simulink model "robot_locomotion_SL_VelTurn"  (R2026a)
settings: Solver=VariableStepAuto  StopTime=tEnd  AbsTol=1e-3  EnableMultiTasking=on
values from neighbouring files (symbols this model uses):
  alb = 0.1    [TunedPIDworkspace.mat]
  albv = 0.2    [TunedPIDworkspace.mat]
  altr = 0.3    [TunedPIDworkspace.mat]
  battery_mass = 0.167    [TunedPIDworkspace.mat]    (also in robot_script_RL_Vel.m; robot_script_RL_VelDual.m; robot_script_RL_VelTurn.m)
  battery_z_pos = -0.035    [TunedPIDworkspace.mat]    (also in robot_script_RL_Vel.m; robot_script_RL_VelDual.m; robot_script_RL_VelTurn.m)
  bypass_b = 0    [TunedPIDworkspace.mat]
  bypass_bi = 0    [TunedPIDworkspace.mat]
  bypass_bp = 1    [TunedPIDworkspace.mat]
  bypass_bv = 0    [TunedPIDworkspace.mat]
  fftr = 0    [TunedPIDworkspace.mat]
  ffv = 7    [TunedPIDworkspace.mat]
  Kpb = -0.55    [TunedPIDworkspace.mat]
  kpbp = 1.4    [TunedPIDworkspace.mat]
  Kpbv = -2    [TunedPIDworkspace.mat]
  Kptr = 1    [TunedPIDworkspace.mat]
  kpv = 10    [TunedPIDworkspace.mat]
  mass_left = 0.325    [TunedPIDworkspace.mat]    (also in robot_script_RL_Vel.m; robot_script_RL_VelDual.m; robot_script_RL_VelTurn.m)
  maxV = 10    [TunedPIDworkspace.mat]    (also in robot_script_RL_Vel.m; robot_script_RL_VelDual.m; robot_script_RL_VelTurn.m)
  motor_z_pos = -0.022    [TunedPIDworkspace.mat]    (also in robot_script_RL_Vel.m; robot_script_RL_VelDual.m; robot_script_RL_VelTurn.m)
  N = size(data, 1)    [robot_script_PIDvsNN.m]
  pcb_mass = 0.098    [TunedPIDworkspace.mat]    (also in robot_script_RL_Vel.m; robot_script_RL_VelDual.m; robot_script_RL_VelTurn.m)
  robot_width = 0.15    [TunedPIDworkspace.mat]    (also in robot_script_RL_Vel.m; robot_script_RL_VelDual.m; robot_script_RL_VelTurn.m)
  s = tf('s')    [robot_script_PIDvsNN.m]    (also in robot_script_RL_Vel.m; robot_script_RL_VelDual.m; robot_script_RL_VelTurn.m)
  taubd = 0.15    [TunedPIDworkspace.mat]
  taubi = 0.1    [TunedPIDworkspace.mat]
  taubii = 0.1    [TunedPIDworkspace.mat]
  taubp = 100000    [TunedPIDworkspace.mat]
  taubvd = 0.6    [TunedPIDworkspace.mat]
  taubvf = 0.01    [TunedPIDworkspace.mat]
  taubvi = 1    [TunedPIDworkspace.mat]
  tautrd = 0.22    [TunedPIDworkspace.mat]
  tautri = 0.1    [TunedPIDworkspace.mat]
  tauvi = 0.043    [TunedPIDworkspace.mat]
  vel_bp = 0.4    [TunedPIDworkspace.mat]
  Y = 20*log10(abs(fft(data)))    [robot_script_PIDvsNN.m]
undefined symbols (not defined in the file or in its folder): net_trained, X, Z
libraries: sm_lib x39, fl_lib x16, nesl_utility x15, ee_lib x4, dlconvfclib x3, dlactivationlib x3, dlutilitylib x1, sharedtransform x1
(part 1 of 2)
settings Model: Creator=chr  LastModifiedBy=emil
settings SimscapeCC: SimscapeNominalValues="[{\"value\":\"1\",\"unit\":\"A\"},{\"value\":\"1\",\"unit\":\"bar\"},{\"value\":\"1\",\"unit\":\"cm^2\"},{\"value\":\"1\",\"unit\":\"cm^3/s\"},{\"value\":\"1\",\"unit\":\"kJ/kg\"},{\"value\":\"1\",\"unit\":\"kW\"},{\"value\":\"1\",\"unit\":\"l\"},{\"value\":\"1\",\"unit\":\"N\"},{\"value\":\"1\",\"unit\":\"N*m\"},{\"value\":\"1\",\"unit\":\"V\"}]"  SimscapeLogSimulationStatistics=on
settings ExplorerConfigSet: SimMechanicsOpenEditorOnUpdate=off
settings ExplorerConfigSet: InternalSimMechanicsExplorerSettings=|
  | <ExplorerConfiguration>
  | 
  |   <canonicalview>default</canonicalview>
  | 
  |   <TilePanel>
  |     <TileInfo>
  |       <Tiles Columns="1" Count="1" Height="704" Rows="1" Width="1078">
  |         <Row Weight="1"/>
  |         <Column Weight="1"/>
  |         <Tile Height="1" Width="1" X="0" Y="0"/>
  |       </Tiles>
  |     </TileInfo>
  |     <SceneInfo>
  |       <SceneViewer>
  |         <IsThisViewStd>
  |           <IsStandardView>off</IsStandardView>
  |           <StandardViewName>Front</StandardViewName>
  |         </IsThisViewStd>
  |         <BGColor>
  |           <R>1</R>
  |           <G>1</G>
  |           <B>1</B>
  |           <A>1</A>
  |         </BGColor>
  |         <Camera>
  |           <DoPerspective>off</DoPerspective>
  |           <Position>
  |             <X>48.876368132250072</X>
  |             <Y>-48.984454841396008</Y>
  |             <Z>49.183620508129628</Z>
  |           </Position>
  |           <Center>
  |             <X>-0.11465636167667981</X>
  |             <Y>0.006569652530743042</Y>
  |             <Z>0.19259601420287537</Z>
  |           </Center>
  |           <Up>
  |             <X>-0.40824829046386307</X>
  |             <Y>0.40824829046386307</Y>
  |             <Z>0.81649658092772615</Z>
  |           </Up>
  |           <XLim>2.040943635816892</XLim>
  |           <YLim>2.040943635816892</YLim>
  |           <ViewLimDist>0.01</ViewLimDist>
  |         </Camera>
  |       </SceneViewer>
  |     </SceneInfo>
  |   </TilePanel>
  | 
  |   <MechEditorPanel>
  |     <GfxPanelCameraMap/>
  |     <Cameras/>
  |     <VideoCreator>
  |       <IncludeTiles>All</IncludeTiles>
  |       <IncludeTime>on</IncludeTime>
  |       <IncludeWorldFrame>off</IncludeWorldFrame>
  |       <PlaybackSpeedRatio>1</PlaybackSpeedRatio>
  |       <FrameRate>30</FrameRate>
  |       <FrameSize>auto</FrameSize>
  |       <VideoFormat>UncompressedAVI</VideoFormat>
  |     </VideoCreator>
  |   </MechEditorPanel>
  | 
  |   <PlaybackSettings>
  |     <PlaybackSpeedFactor>4</PlaybackSpeedFactor>
  |   </PlaybackSettings>
  | 
  | </ExplorerConfiguration>

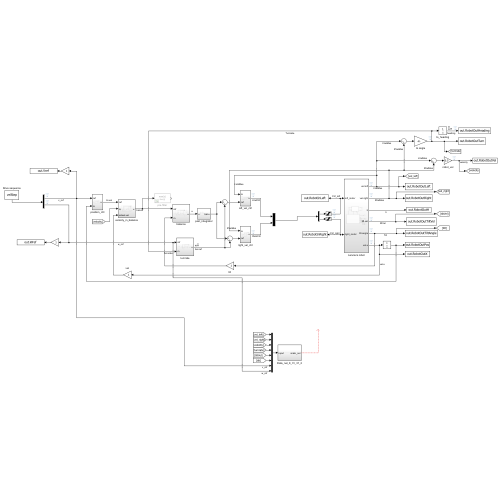
[thumbnail: Simulink's stored preview of the top-level diagram]
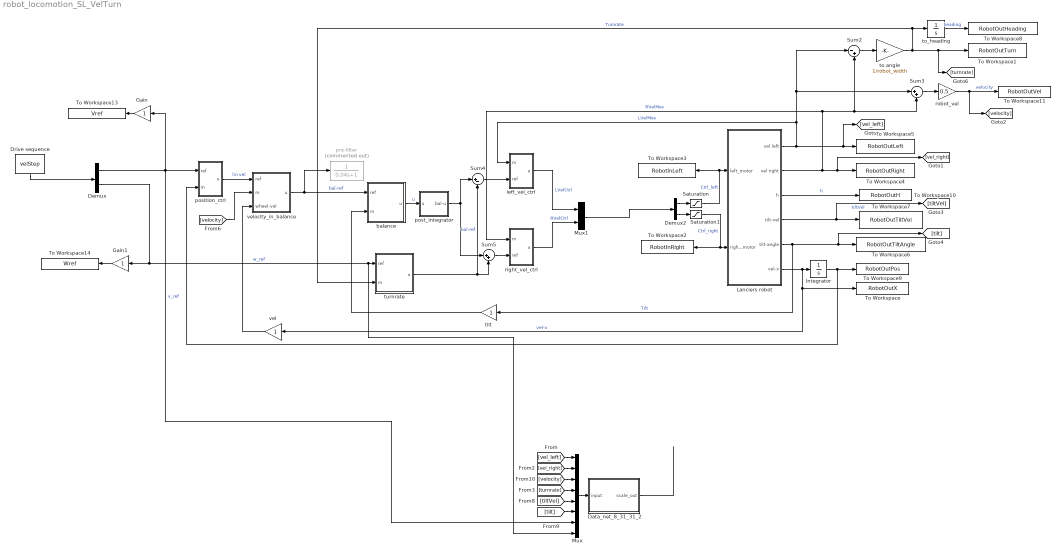
== system robot_locomotion_SL_VelTurn ==
  Data_net_8_31_31_2 : Subsystem
  Demux : Demux  Outputs=2
  Demux2 : Demux  Outputs=2
  Drive sequence : FromWorkspace  VariableName=velStep  Interpolate=off  OutputAfterFinalValue=Setting to zero
  Gain : Gain
  Gain1 : Gain
  Integrator : Integrator
  Lanciers robot : Subsystem
  Mux : Mux  Inputs=8
  Mux1 : Mux  Inputs=2
  Saturation : Saturate  UpperLimit=maxV  LowerLimit=-maxV
  Saturation1 : Saturate  UpperLimit=maxV  LowerLimit=-maxV
  Sum2 : Sum  Inputs=|-+
  Sum3 : Sum  Inputs=|++
  Sum4 : Sum  Inputs=|+-
  Sum5 : Sum  Inputs=|++
  To Workspace : ToWorkspace  VariableName=RobotOutX  SaveFormat=Timeseries  SampleTime=-1
  To Workspace1 : ToWorkspace  VariableName=RobotOutTurn  SaveFormat=Timeseries  SampleTime=-1
  To Workspace10 : ToWorkspace  VariableName=RobotOutH  SaveFormat=Timeseries  SampleTime=-1
  To Workspace11 : ToWorkspace  VariableName=RobotOutVel  SaveFormat=Timeseries  SampleTime=-1
  To Workspace13 : ToWorkspace  VariableName=Vref  SaveFormat=Timeseries  SampleTime=-1
  To Workspace14 : ToWorkspace  VariableName=Wref  SaveFormat=Timeseries  SampleTime=-1
  To Workspace2 : ToWorkspace  VariableName=RobotInRight  SaveFormat=Timeseries  SampleTime=-1
  To Workspace3 : ToWorkspace  VariableName=RobotInLeft  SaveFormat=Timeseries  SampleTime=-1
  To Workspace4 : ToWorkspace  VariableName=RobotOutRight  SaveFormat=Timeseries  SampleTime=-1
  To Workspace5 : ToWorkspace  VariableName=RobotOutLeft  SaveFormat=Timeseries  SampleTime=-1
  To Workspace6 : ToWorkspace  VariableName=RobotOutTiltAngle  SaveFormat=Timeseries  SampleTime=-1
  To Workspace7 : ToWorkspace  VariableName=RobotOutTiltVel  SaveFormat=Timeseries  SampleTime=-1
  To Workspace8 : ToWorkspace  VariableName=RobotOutHeading  SaveFormat=Timeseries  SampleTime=-1
  To Workspace9 : ToWorkspace  VariableName=RobotOutPos  SaveFormat=Timeseries  SampleTime=-1
  balance : Subsystem
  left_vel_ctrl : Subsystem
  position_ctrl : Subsystem
  post_integrator : Subsystem
  pre-filter : TransferFcn  Commented=on  Denominator=[0.04 1]
  right_vel_ctrl : Subsystem
  robot_vel : Gain  Gain=0.5
  tilt : Gain
  to angle : Gain  Gain=1/robot_width
  to_heading : Integrator
  turnrate : Subsystem
  vel : Gain
  velocity_in_balance : Subsystem
  wires:
  Drive sequence/1 -> Demux/1
  Sum2/1 -> to angle/1
  Sum3/1 -> robot_vel/1
  robot_vel/1 -> [velocity], To Workspace11/1  "velocity"
  to angle/1 -> [turnrate], To Workspace1/1, to_heading/1, turnrate/2(m)  "Turnrate"
  Lanciers robot/1(vel left) -> [vel_left], To Workspace5/1, Sum2/1, Sum3/1, left_vel_ctrl/1(m)  "LVelMes"
  Lanciers robot/2(vel right) -> Sum3/2, Sum2/2, right_vel_ctrl/1(m), [vel_right], To Workspace4/1  "RVelMes"
  Lanciers robot/5(tilt-angle) -> tilt/1, [tilt], To Workspace6/1  "Tilt"
  Sum4/1 -> left_vel_ctrl/2(ref)
  Sum5/1 -> right_vel_ctrl/2(ref)
  turnrate/1(u) -> Sum4/2, Sum5/2  "bal-ref"
  position_ctrl/1(u) -> velocity_in_balance/1(ref)  "lin vel"
  Demux/2 -> Mux/8, turnrate/1(ref), Gain1/1  "w_ref"
  tilt/1 -> balance/2(m)
  post_integrator/1(bal-u) -> Sum5/1, Sum4/1
  Lanciers robot/6(vel-x) -> vel/1, To Workspace/1, Integrator/1  "vel-x"
  balance/1(u) -> post_integrator/1(u)  "u"
  Lanciers robot/4(tilt-vel) -> [tiltVel], To Workspace7/1  "tiltVel"
  vel/1 -> velocity_in_balance/3(wheel-vel)
  Demux/1 -> position_ctrl/1(ref), Gain/1, Mux/7  "v_ref"
  Integrator/1 -> To Workspace9/1, position_ctrl/2(m)
  to_heading/1 -> To Workspace8/1  "heading"
  velocity_in_balance/1(u) -> pre-filter/1, balance/1(ref)  "bal-ref"
  Lanciers robot/3(h) -> To Workspace10/1  "h"
  Demux2/2 -> Saturation1/1
  Gain/1 -> To Workspace13/1
  Gain1/1 -> To Workspace14/1
  Demux2/1 -> Saturation/1
  Saturation/1 -> To Workspace3/1, Lanciers robot/1(left_motor)  "Ctrl_left"
  Saturation1/1 -> Lanciers robot/2(right_motor), To Workspace2/1  "Ctrl_right"
  right_vel_ctrl/1(u) -> Mux1/2  "RVelCtrl"
  left_vel_ctrl/1(u) -> Mux1/1  "LVelCtrl"
  [velocity] -> velocity_in_balance/2(m)
  [vel_left] -> Mux/1
  [vel_right] -> Mux/2
  Mux/1 -> Data_net_8_31_31_2/1(input)
  [velocity] -> Mux/3
  [turnrate] -> Mux/4
  [tiltVel] -> Mux/5
  [tilt] -> Mux/6
  Mux1/1 -> Demux2/1
  Data_net_8_31_31_2/1(scale_out) -> ?

== system robot_locomotion_SL_VelTurn/Data_net_8_31_31_2 ==
  input : Inport  PortDimensions=[8]
  FC1 : dlconvfclib/Fully Connected Layer  Layer=net_trained.Layers(2)  OutMin=[]  OutMax=[]  WeightsDataTypeStr=Inherit: Inherit via back propagation  WeightsMin=[]  WeightsMax=[]  BiasDataTypeStr=Inherit: Inherit via back propagation  BiasMin=[]  BiasMax=[]  AccumMin=[]  AccumMax=[]  InternalRndMeth=Floor  InternalSaturateOnIntegerOverflow=off  SampleTime=-1
      settings: DataFormat=C
  FC2 : dlconvfclib/Fully Connected Layer  Layer=net_trained.Layers(4)  OutMin=[]  OutMax=[]  WeightsDataTypeStr=Inherit: Inherit via back propagation  WeightsMin=[]  WeightsMax=[]  BiasDataTypeStr=Inherit: Inherit via back propagation  BiasMin=[]  BiasMax=[]  AccumMin=[]  AccumMax=[]  InternalRndMeth=Floor  InternalSaturateOnIntegerOverflow=off  SampleTime=-1
      settings: DataFormat=C
  FC3 : dlconvfclib/Fully Connected Layer  Layer=net_trained.Layers(6)  OutMin=[]  OutMax=[]  WeightsDataTypeStr=Inherit: Inherit via back propagation  WeightsMin=[]  WeightsMax=[]  BiasDataTypeStr=Inherit: Inherit via back propagation  BiasMin=[]  BiasMax=[]  AccumMin=[]  AccumMax=[]  InternalRndMeth=Floor  InternalSaturateOnIntegerOverflow=off  SampleTime=-1
      settings: DataFormat=C
  Relu1 : dlactivationlib/ReLU Layer  OutMin=[]  OutMax=[]  SampleTime=-1
  Relu2 : dlactivationlib/ReLU Layer  OutMin=[]  OutMax=[]  SampleTime=-1
  scale : dlutilitylib/Scaling Layer  Scale=net_trained.Layers(8).Scale  OutMin=[]  OutMax=[]  ScaleDataTypeStr=Inherit: Inherit via back propagation  ScaleMin=[]  ScaleMax=[]  OffsetDataTypeStr=Inherit: Inherit via back propagation  OffsetMin=[]  OffsetMax=[]  AccumMin=[]  AccumMax=[]  InternalRndMeth=Floor  InternalSaturateOnIntegerOverflow=off  SampleTime=-1  Offset=net_trained.Layers(8).Offset
      settings: DataFormat=C
  tanh : dlactivationlib/Tanh Layer  ApproximationMethod=None  OutMin=[]  OutMax=[]  SampleTime=-1
  scale_out : Outport
  wires:
  FC3/1 -> tanh/1
  FC2/1 -> Relu2/1
  tanh/1 -> scale/1
  input/1 -> FC1/1
  Relu2/1 -> FC3/1
  FC1/1 -> Relu1/1
  scale/1 -> scale_out/1
  Relu1/1 -> FC2/1

== system robot_locomotion_SL_VelTurn/Lanciers robot ==
  left_motor : Inport
  right_motor : Inport  Port=2
  Reference Environment : Subsystem
      settings: PortSchema="{\"entries\":[{\"content\":{\"sides\":[{\"content\":{},\"type\":\"ConnectorPlacement.EquallySpacedRectSide\",\"uuid\":\"28536c2c-3acf-4059-bdab-afc711835bc2\"},{\"content\":{\"connectorIds\":[\"Out1\",\"Out2\",\"Out3\",\"Out4\",\"Out5\"],\"side\":\"RIGHT\"},\"type\":\"ConnectorPlacement.EquallySpacedRectSide\",\"uuid\":\"b1b47e0d-84ad-4acc-8fc9-0385fdd57c1d\"},{\"content\":{\"connectorIds\":[\"Out6\",\"LConn1\",\"LConn2\"],\"side\":\"TOP\"},\"type\":\"ConnectorPlacement.EquallySpacedRectSide\",\"uuid\":\"6bbf457b-7959-4bee-a0d8-17cc0e237686\"}]},\"type\":\"ConnectorPlacement.EquallySpacedConnector\",\"uuid\":\"f4fd0483-f2bb-4404-ae11-e9c07fc10f2b\"}],\"packageUris\":[\"http://schema.mathworks.com/mf0/Connector/R2020b\"],\"version\":\"1.0\"}"
  Robot : Subsystem
      settings: PortSchema="{\"entries\":[{\"content\":{\"sides\":[{\"content\":{\"connectorIds\":[\"In1\",\"In2\",\"In3\"]},\"type\":\"ConnectorPlacement.EquallySpacedRectSide\",\"uuid\":\"5a899b80-7bac-4a74-b0d1-ad24c86580e3\"},{\"content\":{\"connectorIds\":[\"Out1\",\"Out2\"],\"side\":\"RIGHT\"},\"type\":\"ConnectorPlacement.EquallySpacedRectSide\",\"uuid\":\"60cad417-51c5-419f-810a-16084ccef033\"},{\"content\":{\"side\":\"TOP\"},\"type\":\"ConnectorPlacement.EquallySpacedRectSide\",\"uuid\":\"760a64fb-dc53-4169-88c1-c789a5010212\"},{\"content\":{\"connectorIds\":[\"RConn1\",\"RConn2\"],\"side\":\"BOTTOM\"},\"type\":\"ConnectorPlacement.EquallySpacedRectSide\",\"uuid\":\"cf7f532b-f075-440e-839e-2e4da8c12517\"}]},\"type\":\"ConnectorPlacement.EquallySpacedConnector\",\"uuid\":\"eeed42c3-d3c5-4ff3-a0f9-0d560bfc408a\"}],\"packageUris\":[\"http://schema.mathworks.com/mf0/Connector/R2020b\"],\"version\":\"1.0\"}"
  Vel+tilt : Scope  NumInputPorts=4
      settings: ActiveDisplayYMinimum=-0.41559  ActiveDisplayYMaximum=0.42248  DataLoggingVariableName=ScopeData2
  vel left : Outport
  vel right : Outport  Port=2
  h : Outport  Port=3
  tilt-vel : Outport  Port=4
  tilt-angle : Outport  Port=5
  vel-x : Outport  Port=6
  wires:
  left_motor/1 -> Robot/1(left_motor)
  Robot/1(vel left) -> vel left/1  "vel left"
  Robot/2(vel right) -> vel right/1  "vel right"
  right_motor/1 -> Robot/2(right_motor)
  Reference Environment/6(damping) -> Robot/3(force)
  Reference Environment/1(heading) -> h/1
  Reference Environment/3(vel-x) -> vel-x/1, Vel+tilt/1  "vel-x"
  Reference Environment/4(tilt) -> tilt-angle/1, Vel+tilt/2  "tilt"
  Reference Environment/5(wy) -> tilt-vel/1, Vel+tilt/3  "tilt-vel"
  Reference Environment/2(roll) -> Vel+tilt/4
  connections:
  Robot/RConn1 -- Reference Environment/LConn1
  Reference Environment/LConn2 -- Robot/RConn2

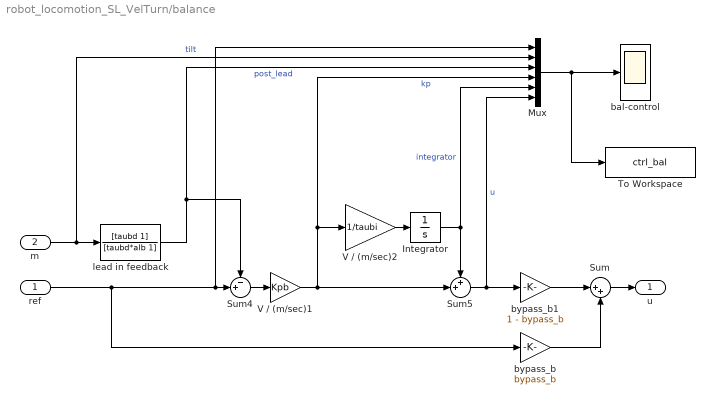
== system robot_locomotion_SL_VelTurn/balance ==
  ref : Inport
  m : Inport  Port=2
  Integrator : Integrator  LimitOutput=on  UpperSaturationLimit=2  LowerSaturationLimit=-2
  Mux : Mux  Inputs=6
  Sum : Sum  Inputs=|++
  Sum4 : Sum  Inputs=-+|
  Sum5 : Sum  Inputs=++|
  To Workspace : ToWorkspace  VariableName=ctrl_bal  SaveFormat=Timeseries  SampleTime=-1
  V / (m/sec)1 : Gain  Gain=Kpb
  V / (m/sec)2 : Gain  Gain=1/taubi
  bal-control : Scope
      settings: ActiveDisplayYMinimum=-0.56215284294128687  ActiveDisplayYMaximum=0.55963423576340021  DataLoggingVariableName=ScopeData3
  bypass_b : Gain  Gain=bypass_b
  bypass_b1 : Gain  Gain=1 - bypass_b
  lead in feedback : TransferFcn  Numerator=[taubd 1]  Denominator=[taubd*alb 1]
  u : Outport
  wires:
  m/1 -> Mux/2, lead in feedback/1  "tilt"
  Sum4/1 -> V / (m/sec)1/1
  V / (m/sec)1/1 -> Mux/4, V / (m/sec)2/1, Sum5/2  "kp"
  Integrator/1 -> Mux/5, Sum5/1  "integrator"
  V / (m/sec)2/1 -> Integrator/1
  lead in feedback/1 -> Mux/3, Sum4/1  "post_lead"
  Sum5/1 -> Mux/6, bypass_b1/1  "u"
  ref/1 -> bypass_b/1, Mux/1, Sum4/2
  Sum/1 -> u/1
  bypass_b1/1 -> Sum/1
  bypass_b/1 -> Sum/2
  Mux/1 -> To Workspace/1, bal-control/1

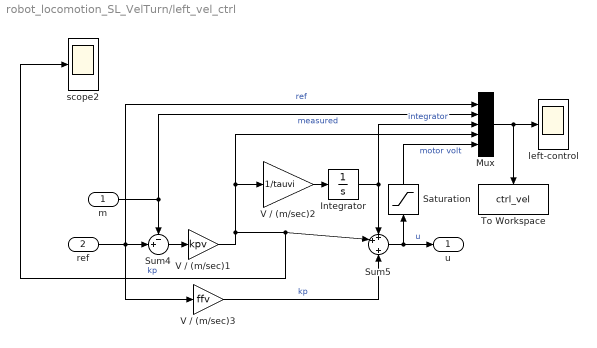
== system robot_locomotion_SL_VelTurn/left_vel_ctrl ==
  m : Inport
  ref : Inport  Port=2
  Integrator : Integrator  LimitOutput=on  UpperSaturationLimit=maxV  LowerSaturationLimit=-maxV
  Mux : Mux  Inputs=5
  Saturation : Saturate  UpperLimit=maxV  LowerLimit=-maxV
  Sum4 : Sum  Inputs=-+|
  Sum5 : Sum  Inputs=++|+
  To Workspace : ToWorkspace  VariableName=ctrl_vel  SaveFormat=Timeseries  SampleTime=-1
  V / (m/sec)1 : Gain  Gain=kpv
  V / (m/sec)2 : Gain  Gain=1/tauvi
  V / (m/sec)3 : Gain  Gain=ffv
  left-control : Scope
      settings: ActiveDisplayYMinimum=-5.5968206382847665  ActiveDisplayYMaximum=12.094205724056652  DataLoggingVariableName=ScopeData3
  scope2 : Scope
      settings: ActiveDisplayYMinimum=-1.0107410448004606  ActiveDisplayYMaximum=1.3463203831097874
  u : Outport
  wires:
  V / (m/sec)2/1 -> Integrator/1
  Integrator/1 -> Mux/3, Sum5/1  "integrator"
  ref/1 -> Sum4/2, Mux/1, V / (m/sec)3/1  "ref"
  V / (m/sec)1/1 -> scope2/1, Sum5/2, Mux/4, V / (m/sec)2/1  "kp"
  Sum5/1 -> Saturation/1, u/1  "u"
  Sum4/1 -> V / (m/sec)1/1
  m/1 -> Mux/2, Sum4/1  "measured"
  V / (m/sec)3/1 -> Sum5/3  "kp"
  Mux/1 -> left-control/1, To Workspace/1
  Saturation/1 -> Mux/5  "motor volt"

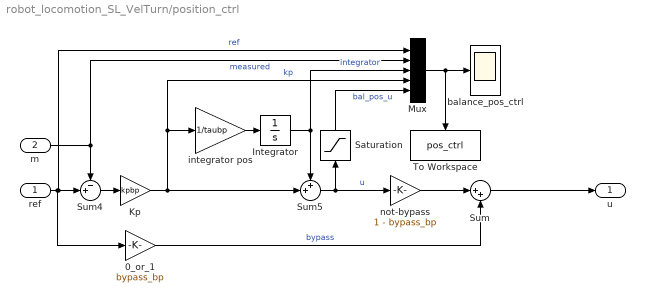
== system robot_locomotion_SL_VelTurn/position_ctrl ==
  ref : Inport
  m : Inport  Port=2
  0_or_1 : Gain  Gain=bypass_bp
  Integrator : Integrator  LimitOutput=on  UpperSaturationLimit=maxV  LowerSaturationLimit=-maxV
  Kp : Gain  Gain=kpbp
  Mux : Mux  Inputs=5
  Saturation : Saturate  UpperLimit=vel_bp  LowerLimit=-vel_bp
  Sum : Sum  Inputs=|++
  Sum4 : Sum  Inputs=-+|
  Sum5 : Sum  Inputs=++|
  To Workspace : ToWorkspace  VariableName=pos_ctrl  SaveFormat=Timeseries  SampleTime=-1
  balance_pos_ctrl : Scope
      settings: ActiveDisplayYMinimum=-5.5968206382847665  ActiveDisplayYMaximum=12.094205724056652  DataLoggingVariableName=ScopeData3
  integrator pos : Gain  Gain=1/taubp
  not-bypass : Gain  Gain=1 - bypass_bp
  u : Outport
  wires:
  Saturation/1 -> Mux/5  "bal_pos_u"
  Mux/1 -> To Workspace/1, balance_pos_ctrl/1
  0_or_1/1 -> Sum/2  "bypass"
  m/1 -> Sum4/1, Mux/2  "measured"
  Sum4/1 -> Kp/1
  Sum5/1 -> Saturation/1, not-bypass/1  "u"
  Kp/1 -> integrator pos/1, Mux/4, Sum5/2  "kp"
  ref/1 -> Sum4/2, Mux/1, 0_or_1/1  "ref"
  Integrator/1 -> Sum5/1, Mux/3  "integrator"
  integrator pos/1 -> Integrator/1
  Sum/1 -> u/1
  not-bypass/1 -> Sum/1

== system robot_locomotion_SL_VelTurn/post_integrator ==
  u : Inport
  Integrator1 : Integrator  LimitOutput=on  UpperSaturationLimit=1  LowerSaturationLimit=-1
  Sum : Sum  Inputs=|++
  Sum1 : Sum  Inputs=++|
  V / (m/sec)3 : Gain  Gain=1/taubii
  bypass_bi : Gain  Gain=bypass_bi
  bypass_bi1 : Gain  Gain=1 - bypass_bi
  bal-u : Outport
  wires:
  Integrator1/1 -> Sum1/1  "integrator"
  V / (m/sec)3/1 -> Integrator1/1
  Sum1/1 -> bypass_bi1/1  "bal-u"
  u/1 -> V / (m/sec)3/1, bypass_bi/1, Sum1/2
  bypass_bi/1 -> Sum/2
  bypass_bi1/1 -> Sum/1
  Sum/1 -> bal-u/1

== system robot_locomotion_SL_VelTurn/right_vel_ctrl ==
  m : Inport
  ref : Inport  Port=2
  Integrator : Integrator  LimitOutput=on  UpperSaturationLimit=maxV  LowerSaturationLimit=-maxV
  Sum4 : Sum  Inputs=-+|
  Sum5 : Sum  Inputs=++|+
  V / (m/sec)1 : Gain  Gain=kpv
  V / (m/sec)2 : Gain  Gain=1/tauvi
  V / (m/sec)3 : Gain  Gain=ffv
  left vel ctrl : Scope  NumInputPorts=3
      settings: ActiveDisplayYMinimum=-14.34853  ActiveDisplayYMaximum=96.85184  DataLoggingVariableName=ScopeData4
  u : Outport
  wires:
  m/1 -> Sum4/1
  Sum4/1 -> V / (m/sec)1/1
  Sum5/1 -> left vel ctrl/3, u/1  "u"
  V / (m/sec)1/1 -> left vel ctrl/1, V / (m/sec)2/1, Sum5/2  "kp"
  ref/1 -> V / (m/sec)3/1, Sum4/2
  Integrator/1 -> left vel ctrl/2, Sum5/1  "int"
  V / (m/sec)2/1 -> Integrator/1
  V / (m/sec)3/1 -> Sum5/3  "kp"

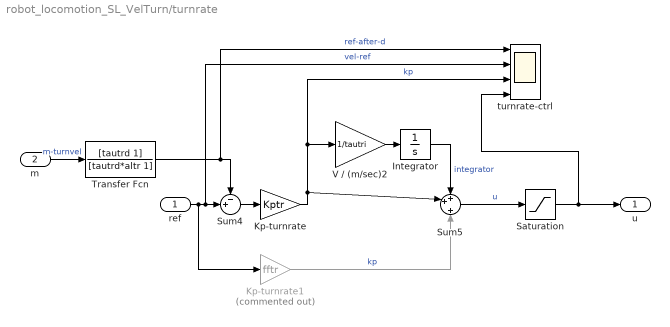
== system robot_locomotion_SL_VelTurn/turnrate ==
  ref : Inport
  m : Inport  Port=2
  Integrator : Integrator
  Kp-turnrate : Gain  Gain=Kptr
  Kp-turnrate1 : Gain  Commented=on  Gain=fftr
  Saturation : Saturate  UpperLimit=0.15  LowerLimit=-0.15
  Sum4 : Sum  Inputs=-+|
  Sum5 : Sum  Inputs=++|+
  Transfer Fcn : TransferFcn  Numerator=[tautrd 1]  Denominator=[tautrd*altr 1]
  V / (m/sec)2 : Gain  Gain=1/tautri
  turnrate-ctrl : Scope  NumInputPorts=4
      settings: ActiveDisplayYMinimum=-0.01795  ActiveDisplayYMaximum=0.36111  DataLoggingVariableName=ScopeData3
  u : Outport
  wires:
  Transfer Fcn/1 -> turnrate-ctrl/1, Sum4/1  "ref-after-d"
  m/1 -> Transfer Fcn/1  "m-turnvel"
  Sum4/1 -> Kp-turnrate/1
  Kp-turnrate/1 -> turnrate-ctrl/3, V / (m/sec)2/1, Sum5/2  "kp"
  ref/1 -> Kp-turnrate1/1, turnrate-ctrl/2, Sum4/2  "vel-ref"
  Integrator/1 -> Sum5/1  "integrator"
  V / (m/sec)2/1 -> Integrator/1
  Sum5/1 -> Saturation/1  "u"
  Kp-turnrate1/1 -> Sum5/3  "kp"
  Saturation/1 -> turnrate-ctrl/4, u/1

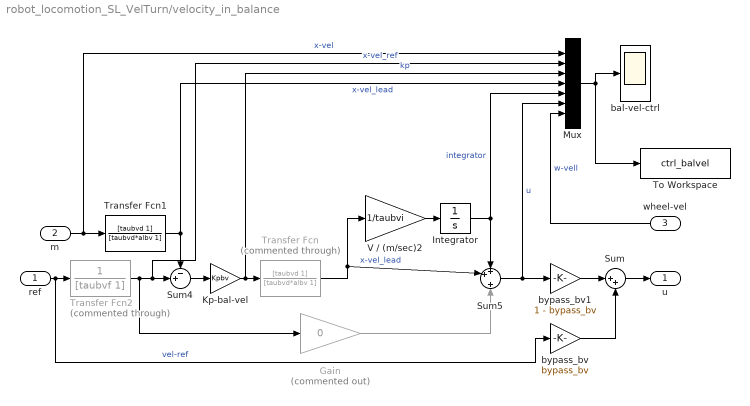
== system robot_locomotion_SL_VelTurn/velocity_in_balance ==
  ref : Inport
  m : Inport  Port=2
  wheel-vel : Inport  Port=3
  Gain : Gain  Commented=on  Gain=0
  Integrator : Integrator  LimitOutput=on  UpperSaturationLimit=2  LowerSaturationLimit=-2
  Kp-bal-vel : Gain  Gain=Kpbv
  Mux : Mux  Inputs=7
  Sum : Sum  Inputs=|++
  Sum4 : Sum  Inputs=-+|
  Sum5 : Sum  Inputs=++|+
  To Workspace : ToWorkspace  VariableName=ctrl_balvel  SaveFormat=Timeseries  SampleTime=-1
  Transfer Fcn : TransferFcn  Commented=through  Numerator=[taubvd 1]  Denominator=[taubvd*albv 1]
  Transfer Fcn1 : TransferFcn  Numerator=[taubvd 1]  Denominator=[taubvd*albv 1]
  Transfer Fcn2 : TransferFcn  Commented=through  Denominator=[taubvf 1]
  V / (m/sec)2 : Gain  Gain=1/taubvi
  bal-vel-ctrl : Scope
      settings: ActiveDisplayYMinimum=-1.5650191081710629  ActiveDisplayYMaximum=1.1450603981933434  DataLoggingVariableName=ScopeData3
  bypass_bv : Gain  Gain=bypass_bv
  bypass_bv1 : Gain  Gain=1 - bypass_bv
  u : Outport
  wires:
  Sum5/1 -> Mux/6, bypass_bv1/1  "u"
  V / (m/sec)2/1 -> Integrator/1
  Integrator/1 -> Mux/5, Sum5/1  "integrator"
  ref/1 -> bypass_bv/1, Transfer Fcn2/1  "vel-ref"
  Kp-bal-vel/1 -> Mux/3, Transfer Fcn/1  "kp"
  Sum4/1 -> Kp-bal-vel/1
  m/1 -> Transfer Fcn1/1, Mux/1  "x-vel"
  bypass_bv/1 -> Sum/2
  bypass_bv1/1 -> Sum/1
  Sum/1 -> u/1
  Mux/1 -> bal-vel-ctrl/1, To Workspace/1
  Transfer Fcn/1 -> Sum5/2, V / (m/sec)2/1  "x-vel_lead"
  Transfer Fcn1/1 -> Mux/4, Sum4/1  "x-vel_lead"
  Transfer Fcn2/1 -> Gain/1, Mux/2, Sum4/2  "x-vel_ref"
  wheel-vel/1 -> Mux/7  "w-vell"
  Gain/1 -> Sum5/3

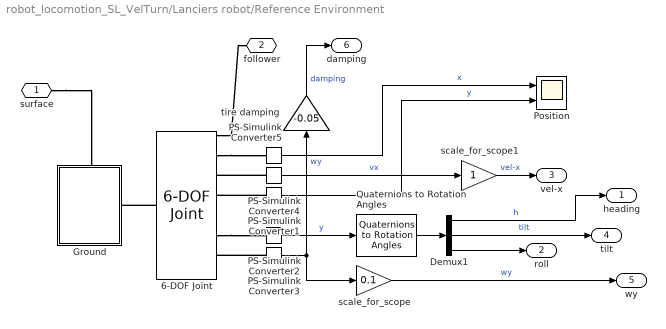
== system robot_locomotion_SL_VelTurn/Lanciers robot/Reference Environment ==
  6-DOF Joint : sm_lib/Joints/6-DOF Joint  JointMode=Normal  CompositeWrenchDir=FollowerOnBase  CompositeWrenchFrame=BaseFrame  SenseConstraintForce=off  SenseConstraintTorque=off  SenseTotalForce=off  SenseTotalTorque=off  PxPositionTargetSpecify=off  PxPositionTargetPriority=High  PxPositionTargetValue=0  PxPositionTargetValueUnits=m  PxVelocityTargetSpecify=off  PxVelocityTargetPriority=High  PxVelocityTargetValue=0  PxVelocityTargetValueUnits=m/s  PxEquilibriumPosition=0  PxEquilibriumPositionUnits=m  PxSpringStiffness=0  PxSpringStiffnessUnits=N/m  PxDampingCoefficient=0  PxDampingCoefficientUnits=N/(m/s)  PxLowerLimitSpecify=off  PxLowerLimitBound=-1  PxLowerLimitBoundUnits=m  PxLowerLimitStiffness=1e6  PxLowerLimitStiffnessUnits=N/m  PxLowerLimitDamping=1e3  PxLowerLimitDampingUnits=N/(m/s)  PxLowerLimitTransitionRegionWidth=1e-4  PxLowerLimitTransitionRegionWidthUnits=m  PxUpperLimitSpecify=off  PxUpperLimitBound=1  PxUpperLimitBoundUnits=m  PxUpperLimitStiffness=1e6  PxUpperLimitStiffnessUnits=N/m  PxUpperLimitDamping=1e3  PxUpperLimitDampingUnits=N/(m/s)  PxUpperLimitTransitionRegionWidth=1e-4  PxUpperLimitTransitionRegionWidthUnits=m  PxTorqueActuationMode=NoTorque  PxMotionActuationMode=ComputedMotion  PxSensePosition=on  PxSenseVelocity=on  PxSenseAcceleration=off  PxSenseTorqueForce=off  PxSenseLowerLimitTorqueForce=off  PxSenseUpperLimitTorqueForce=off  PyPositionTargetSpecify=off  PyPositionTargetPriority=High  PyPositionTargetValue=0  PyPositionTargetValueUnits=m  PyVelocityTargetSpecify=off  PyVelocityTargetPriority=High  PyVelocityTargetValue=0  PyVelocityTargetValueUnits=m/s  PyEquilibriumPosition=0  PyEquilibriumPositionUnits=m  PySpringStiffness=0  PySpringStiffnessUnits=N/m  PyDampingCoefficient=0  PyDampingCoefficientUnits=N/(m/s)  PyLowerLimitSpecify=off  PyLowerLimitBound=-1  PyLowerLimitBoundUnits=m  PyLowerLimitStiffness=1e6  PyLowerLimitStiffnessUnits=N/m  PyLowerLimitDamping=1e3  PyLowerLimitDampingUnits=N/(m/s)  PyLowerLimitTransitionRegionWidth=1e-4  PyLowerLimitTransitionRegionWidthUnits=m  PyUpperLimitSpecify=off  PyUpperLimitBound=1  PyUpperLimitBoundUnits=m  PyUpperLimitStiffness=1e6  PyUpperLimitStiffnessUnits=N/m  PyUpperLimitDamping=1e3  PyUpperLimitDampingUnits=N/(m/s)  PyUpperLimitTransitionRegionWidth=1e-4  PyUpperLimitTransitionRegionWidthUnits=m  PyTorqueActuationMode=NoTorque  PyMotionActuationMode=ComputedMotion  PySensePosition=on  PySenseVelocity=on  PySenseAcceleration=off  PySenseTorqueForce=off  PySenseLowerLimitTorqueForce=off  PySenseUpperLimitTorqueForce=off  PzPositionTargetSpecify=off  PzPositionTargetPriority=High  PzPositionTargetValue=0  PzPositionTargetValueUnits=m  PzVelocityTargetSpecify=off  PzVelocityTargetPriority=High  PzVelocityTargetValue=0  PzVelocityTargetValueUnits=m/s  PzEquilibriumPosition=0  PzEquilibriumPositionUnits=m  PzSpringStiffness=0  PzSpringStiffnessUnits=N/m  PzDampingCoefficient=0  PzDampingCoefficientUnits=N/(m/s)  PzLowerLimitSpecify=off  PzLowerLimitBound=-1  PzLowerLimitBoundUnits=m  PzLowerLimitStiffness=1e6  PzLowerLimitStiffnessUnits=N/m  PzLowerLimitDamping=1e3  PzLowerLimitDampingUnits=N/(m/s)  PzLowerLimitTransitionRegionWidth=1e-4  PzLowerLimitTransitionRegionWidthUnits=m  PzUpperLimitSpecify=off  PzUpperLimitBound=1  PzUpperLimitBoundUnits=m  PzUpperLimitStiffness=1e6  PzUpperLimitStiffnessUnits=N/m  PzUpperLimitDamping=1e3  PzUpperLimitDampingUnits=N/(m/s)  PzUpperLimitTransitionRegionWidth=1e-4  PzUpperLimitTransitionRegionWidthUnits=m  PzTorqueActuationMode=NoTorque  PzMotionActuationMode=ComputedMotion  PzSensePosition=off  PzSenseVelocity=off  PzSenseAcceleration=off  PzSenseTorqueForce=off  PzSenseLowerLimitTorqueForce=off  PzSenseUpperLimitTorqueForce=off  SphPositionTargetSpecify=off  SphPositionTargetPriority=High  SphPositionTargetRotationMethod=None  SphPositionTargetFollAlignAxisA=+X  SphPositionTargetBaseAlignAxisA=+Y  SphPositionTargetFollAlignAxisB=+Y  SphPositionTargetBaseAlignAxisB=+Z  SphPositionTargetRotationStandardAxis=+Z  SphPositionTargetRotationAngle=0.0  SphPositionTargetRotationAngleUnits=deg  SphPositionTargetRotationArbitraryAxis=[0 0 1]  SphPositionTargetRotationSequenceAxes=FollowerAxes  SphPositionTargetRotationSequence=XYX  SphPositionTargetRotationSequenceAngles=[0 0 0]  SphPositionTargetRotationSequenceAnglesUnits=deg  SphPositionTargetRotationMatrix=[1 0 0; 0 1 0; 0 0 1]  SphPositionTargetQuaternion=[1 0 0 0]  SphVelocityTargetSpecify=off  SphVelocityTargetPriority=High  SphVelocityTargetValue=[0 0 0]  SphVelocityTargetValueUnits=deg/s  SphVelocityTargetInFollowerFrame=on  SphEqPosRotationMethod=None  SphEqPosFollAlignAxisA=+X  SphEqPosBaseAlignAxisA=+Y  SphEqPosFollAlignAxisB=+Y  SphEqPosBaseAlignAxisB=+Z  SphEqPosRotationStandardAxis=+Z  SphEqPosRotationAngle=0.0  SphEqPosRotationAngleUnits=deg  SphEqPosRotationArbitraryAxis=[0 0 1]  SphEqPosRotationSequenceAxes=FollowerAxes  SphEqPosRotationSequence=XYX  SphEqPosRotationSequenceAngles=[0 0 0]  SphEqPosRotationSequenceAnglesUnits=deg  SphEqPosRotationMatrix=[1 0 0; 0 1 0; 0 0 1]  SphEqPosQuaternion=[1 0 0 0]  SphSpringStiffness=0  SphSpringStiffnessUnits=N*m/deg  SphDampingCoefficient=0  SphDampingCoefficientUnits=N*m/(deg/s)  SphLowerLimitSpecify=off  SphLowerLimitBound=15  SphLowerLimitBoundUnits=deg  SphLowerLimitStiffness=1e4  SphLowerLimitStiffnessUnits=N*m/deg  SphLowerLimitDamping=10  SphLowerLimitDampingUnits=N*m/(deg/s)  SphLowerLimitTransitionRegionWidth=0.1  SphLowerLimitTransitionRegionWidthUnits=deg  SphUpperLimitSpecify=off  SphUpperLimitBound=45  SphUpperLimitBoundUnits=deg  SphUpperLimitStiffness=1e4  SphUpperLimitStiffnessUnits=N*m/deg  SphUpperLimitDamping=10  SphUpperLimitDampingUnits=N*m/(deg/s)  SphUpperLimitTransitionRegionWidth=0.1  SphUpperLimitTransitionRegionWidthUnits=deg  SphTorqueActuationMode=NoTorque  SphActuateTorqueX=off  SphActuateTorqueY=off  SphActuateTorqueZ=off  SphActuateTorque=off  SphActuationFrame=BaseFrame  SphSensePosition=on  SphSenseVelocityX=off  SphSenseVelocityY=on  SphSenseVelocityZ=on  SphSenseVelocity=off  SphSenseAccelerationX=off  SphSenseAccelerationY=off  SphSenseAccelerationZ=off  SphSenseAcceleration=off  SphSenseLowerLimitTorqueMag=off  SphSenseUpperLimitTorqueMag=off  SphSensingFrame=BaseFrame
  Demux1 : Demux  Outputs=3
  Ground : Subsystem
      settings: PortSchema="{\"entries\":[{\"content\":{\"sides\":[{\"content\":{\"connectorIds\":[\"LConn1\"]},\"type\":\"ConnectorPlacement.EquallySpacedRectSide\",\"uuid\":\"7eef4dea-7609-4788-a85a-c84ffa69f19a\"},{\"content\":{\"side\":\"RIGHT\"},\"type\":\"ConnectorPlacement.EquallySpacedRectSide\",\"uuid\":\"e92c1246-1c8b-41a9-8b16-f2f858e0f641\"},{\"content\":{\"connectorIds\":[\"LConn2\"],\"side\":\"TOP\"},\"type\":\"ConnectorPlacement.EquallySpacedRectSide\",\"uuid\":\"82c7f900-0ee0-48a7-aa06-93a152edf391\"},{\"content\":{\"side\":\"BOTTOM\"},\"type\":\"ConnectorPlacement.EquallySpacedRectSide\",\"uuid\":\"9e84da80-f719-4480-b7c4-b32f809bd4ff\"}]},\"type\":\"ConnectorPlacement.EquallySpacedConnector\",\"uuid\":\"a7b1ed51-00a2-4ab2-b1e1-05c20ce69010\"}],\"packageUris\":[\"http://schema.mathworks.com/mf0/Connector/R2020b\"],\"version\":\"1.0\"}"
  PS-Simulink Converter{1..5} (5 alike) : nesl_utility/PS-Simulink Converter  PhysicalDomain=network_engine_domain  SubClassName=ps_output  LeftPortType=input  RightPortType=output  PseudoPeriodic=off  Frequencies=[]  VectorFormat=inherit  Unit=inherit  AffineConversion=off
  Position : Scope  NumInputPorts=2
      settings: ActiveDisplayYMinimum=-0.17986  ActiveDisplayYMaximum=1.61876
  Quaternions to Rotation Angles : sharedtransform/Quaternions to Rotation Angles  rotationOrder=ZYX  aMode=aMode
  scale_for_scope : Gain  Gain=0.1
  scale_for_scope1 : Gain
  tire damping : Gain  Gain=-0.05
  surface : PMIOPort  Side=Left
  follower : PMIOPort  Port=2  Side=Left
  heading : Outport
  roll : Outport  Port=2
  vel-x : Outport  Port=3
  tilt : Outport  Port=4
  wy : Outport  Port=5
  damping : Outport  Port=6
  wires:
  PS-Simulink Converter5/1 -> Position/1  "x"
  Quaternions to Rotation Angles/1 -> Demux1/1
  scale_for_scope/1 -> wy/1  "wy"
  PS-Simulink Converter1/1 -> Position/2  "y"
  Demux1/3 -> roll/1
  tire damping/1 -> damping/1  "damping"
  Demux1/2 -> tilt/1  "tilt"
  PS-Simulink Converter2/1 -> Quaternions to Rotation Angles/1  "y"
  scale_for_scope1/1 -> vel-x/1  "vel-x"
  PS-Simulink Converter3/1 -> scale_for_scope/1, tire damping/1  "wy"
  Demux1/1 -> heading/1  "h"
  PS-Simulink Converter4/1 -> scale_for_scope1/1  "vx"
  connections:
  6-DOF Joint/RConn6 -- PS-Simulink Converter2/LConn1
  surface/RConn1 -- Ground/LConn1
  PS-Simulink Converter4/LConn1 -- 6-DOF Joint/RConn3
  6-DOF Joint/RConn1 -- follower/RConn1
  PS-Simulink Converter1/LConn1 -- 6-DOF Joint/RConn4
  PS-Simulink Converter3/LConn1 -- 6-DOF Joint/RConn7
  6-DOF Joint/LConn1 -- Ground/LConn2
  6-DOF Joint/RConn2 -- PS-Simulink Converter5/LConn1

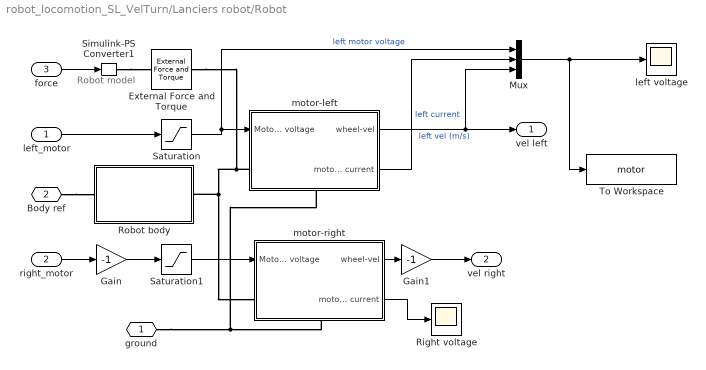
== system robot_locomotion_SL_VelTurn/Lanciers robot/Robot ==
  note: Robot model
  left_motor : Inport
  right_motor : Inport  Port=2
  force : Inport  Port=3
  External Force and Torque : sm_lib/Forces and Torques/External Force and Torque  EnableForceX=on  EnableForceY=off  EnableForceZ=off  EnableForce=off  ForceResolutionFrame=AttachedFrame  EnableTorqueX=off  EnableTorqueY=off  EnableTorqueZ=off  EnableTorque=off  TorqueResolutionFrame=AttachedFrame
  Gain : Gain  Gain=-1
  Gain1 : Gain  Gain=-1
  Mux : Mux  Inputs=3
  Right voltage : Scope
      settings: ActiveDisplayYMinimum=-0.73730574868191467  ActiveDisplayYMaximum=6.3650813632771177  DataLoggingVariableName=ScopeData5
  Robot body : Subsystem
  Saturation : Saturate  UpperLimit=maxV  LowerLimit=-maxV
  Saturation1 : Saturate  UpperLimit=maxV  LowerLimit=-maxV
  Simulink-PS Converter1 : nesl_utility/Simulink-PS Converter  PhysicalDomain=network_engine_domain  SubClassName=ps_input  LeftPortType=input  RightPortType=output  PseudoPeriodic=off  Frequencies=[]  NoiseDistribution=none  NoiseParameters=[]  Unit=1  AffineConversion=off  FilteringAndDerivatives=provide  SimscapeFilterOrder=1  InputFilterTimeConstant=0.001  UdotUserProvided=0
  To Workspace : ToWorkspace  VariableName=motor  SaveFormat=Timeseries  SampleTime=-1
  left voltage : Scope
      settings: ActiveDisplayYMinimum=-0.73730574868191467  ActiveDisplayYMaximum=6.3650813632771177
  motor-left : Subsystem
      settings: PortSchema="{\"entries\":[{\"content\":{\"sides\":[{\"content\":{\"connectorIds\":[\"In1\",\"LConn1\"]},\"type\":\"ConnectorPlacement.EquallySpacedRectSide\",\"uuid\":\"bc06ab0c-ec37-423f-ad89-e6de7599ff9c\"},{\"content\":{\"connectorIds\":[\"Out1\",\"Out2\"],\"side\":\"RIGHT\"},\"type\":\"ConnectorPlacement.EquallySpacedRectSide\",\"uuid\":\"2c5e0562-173d-41fd-949f-bc39ba05f0ab\"},{\"content\":{\"side\":\"TOP\"},\"type\":\"ConnectorPlacement.EquallySpacedRectSide\",\"uuid\":\"af8143ef-f675-4d04-b4a0-18486ad7b1fb\"},{\"content\":{\"connectorIds\":[\"RConn1\"],\"side\":\"BOTTOM\"},\"type\":\"ConnectorPlacement.EquallySpacedRectSide\",\"uuid\":\"299cf55a-d0c8-4529-9079-bde7a1e7c733\"}]},\"type\":\"ConnectorPlacement.EquallySpacedConnector\",\"uuid\":\"886a683f-1c42-4547-b783-dfd3b966f67e\"}],\"packageUris\":[\"http://schema.mathworks.com/mf0/Connector/R2020b\"],\"version\":\"1.0\"}"
  motor-right : Subsystem
      settings: PortSchema="{\"entries\":[{\"content\":{\"sides\":[{\"content\":{\"connectorIds\":[\"In1\",\"LConn1\"]},\"type\":\"ConnectorPlacement.EquallySpacedRectSide\",\"uuid\":\"bc06ab0c-ec37-423f-ad89-e6de7599ff9c\"},{\"content\":{\"connectorIds\":[\"Out1\",\"Out2\"],\"side\":\"RIGHT\"},\"type\":\"ConnectorPlacement.EquallySpacedRectSide\",\"uuid\":\"2c5e0562-173d-41fd-949f-bc39ba05f0ab\"},{\"content\":{\"side\":\"TOP\"},\"type\":\"ConnectorPlacement.EquallySpacedRectSide\",\"uuid\":\"af8143ef-f675-4d04-b4a0-18486ad7b1fb\"},{\"content\":{\"connectorIds\":[\"RConn1\"],\"side\":\"BOTTOM\"},\"type\":\"ConnectorPlacement.EquallySpacedRectSide\",\"uuid\":\"299cf55a-d0c8-4529-9079-bde7a1e7c733\"}]},\"type\":\"ConnectorPlacement.EquallySpacedConnector\",\"uuid\":\"886a683f-1c42-4547-b783-dfd3b966f67e\"}],\"packageUris\":[\"http://schema.mathworks.com/mf0/Connector/R2020b\"],\"version\":\"1.0\"}"
  ground : PMIOPort  Side=Right
  Body ref : PMIOPort  Port=2  Side=Right
  vel left : Outport
  vel right : Outport  Port=2
  wires:
  right_motor/1 -> Gain/1
  motor-left/1(wheel-vel) -> Mux/3, vel left/1  "left vel (m/s)"
  left_motor/1 -> Saturation/1
  Gain/1 -> Saturation1/1
  Saturation/1 -> Mux/1, motor-left/1(Motor voltage)  "left motor voltage"
  Saturation1/1 -> motor-right/1(Motor voltage)
  motor-right/1(wheel-vel) -> Gain1/1
  force/1 -> Simulink-PS Converter1/1
  Gain1/1 -> vel right/1
  Mux/1 -> To Workspace/1, left voltage/1
  motor-left/2(motor current) -> Mux/2  "left current"
  motor-right/2(motor current) -> Right voltage/1
  connections:
  motor-left/LConn1 -- motor-right/LConn1 -- Robot body/RConn1 -- External Force and Torque/RConn1
  ground/RConn1 -- motor-right/RConn1 -- motor-left/RConn1
  Body ref/RConn1 -- Robot body/LConn1
  Simulink-PS Converter1/RConn1 -- External Force and Torque/LConn1

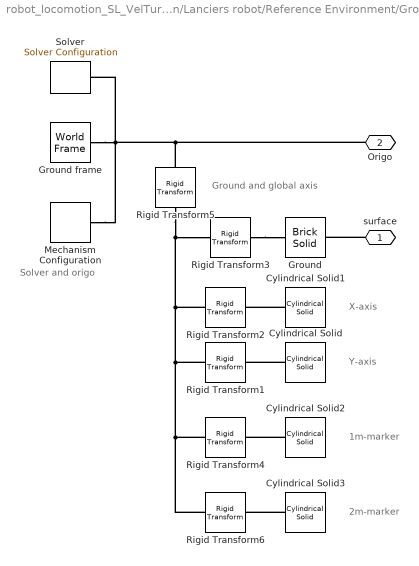
== system robot_locomotion_SL_VelTurn/Lanciers robot/Reference Environment/Ground ==
  note: X-axis
  note: Y-axis
  note: Ground and global axis
  note: Solver and origo
  note: 1m-marker
  note: 2m-marker
  Cylindrical Solid : sm_lib/Body Elements/Cylindrical Solid  CylinderRadius=0.01  CylinderRadiusUnits=m  CylinderLength=2  CylinderLengthUnits=m  ExportEntireGeometry=off  InertiaType=CalculateFromGeometry  BasedOnType=Density  Density=1000  DensityUnits=kg/m^3  Mass=1  MassUnits=kg  CenterOfMass=[0 0 0]  CenterOfMassUnits=m  MomentsOfInertia=[1 1 1]  MomentsOfInertiaUnits=kg*m^2  ProductsOfInertia=[0 0 0]  ProductsOfInertiaUnits=kg*m^2  GraphicType=FromGeometry  MarkerShape=Sphere  MarkerSize=10  GraphicVisPropType=SimpleVisualProperties  GraphicDiffuseColor=[0.6 0.0 0.0]  GraphicOpacity=1.0  GraphicSpecularColor=[0.5 0.5 0.5 1.0]  GraphicAmbientColor=[0.15 0.15 0.15 1.0]  GraphicEmissiveColor=[0.0 0.0 0.0 1.0]  GraphicShininess=75  DoExposeReferenceFrame=on  SerializedFrames=<Frames/>
  Cylindrical Solid1 : sm_lib/Body Elements/Cylindrical Solid  CylinderRadius=0.01  CylinderRadiusUnits=m  CylinderLength=6  CylinderLengthUnits=m  ExportEntireGeometry=off  InertiaType=CalculateFromGeometry  BasedOnType=Density  Density=1000  DensityUnits=kg/m^3  Mass=1  MassUnits=kg  CenterOfMass=[0 0 0]  CenterOfMassUnits=m  MomentsOfInertia=[1 1 1]  MomentsOfInertiaUnits=kg*m^2  ProductsOfInertia=[0 0 0]  ProductsOfInertiaUnits=kg*m^2  GraphicType=FromGeometry  MarkerShape=Sphere  MarkerSize=10  GraphicVisPropType=SimpleVisualProperties  GraphicDiffuseColor=[0.0 0.6 0.0]  GraphicOpacity=1.0  GraphicSpecularColor=[0.5 0.5 0.5 1.0]  GraphicAmbientColor=[0.15 0.15 0.15 1.0]  GraphicEmissiveColor=[0.0 0.0 0.0 1.0]  GraphicShininess=75  DoExposeReferenceFrame=on  SerializedFrames=<Frames/>
  Cylindrical Solid2 : sm_lib/Body Elements/Cylindrical Solid  CylinderRadius=0.003  CylinderRadiusUnits=m  CylinderLength=1  CylinderLengthUnits=m  ExportEntireGeometry=off  InertiaType=CalculateFromGeometry  BasedOnType=Density  Density=1000  DensityUnits=kg/m^3  Mass=1  MassUnits=kg  CenterOfMass=[0 0 0]  CenterOfMassUnits=m  MomentsOfInertia=[1 1 1]  MomentsOfInertiaUnits=kg*m^2  ProductsOfInertia=[0 0 0]  ProductsOfInertiaUnits=kg*m^2  GraphicType=FromGeometry  MarkerShape=Sphere  MarkerSize=10  GraphicVisPropType=SimpleVisualProperties  GraphicDiffuseColor=[0.6 0.0 0.0]  GraphicOpacity=1.0  GraphicSpecularColor=[0.5 0.5 0.5 1.0]  GraphicAmbientColor=[0.15 0.15 0.15 1.0]  GraphicEmissiveColor=[0.0 0.0 0.0 1.0]  GraphicShininess=75  DoExposeReferenceFrame=on  SerializedFrames=<Frames/>
  Cylindrical Solid3 : sm_lib/Body Elements/Cylindrical Solid  CylinderRadius=0.003  CylinderRadiusUnits=m  CylinderLength=1  CylinderLengthUnits=m  ExportEntireGeometry=off  InertiaType=CalculateFromGeometry  BasedOnType=Density  Density=1000  DensityUnits=kg/m^3  Mass=1  MassUnits=kg  CenterOfMass=[0 0 0]  CenterOfMassUnits=m  MomentsOfInertia=[1 1 1]  MomentsOfInertiaUnits=kg*m^2  ProductsOfInertia=[0 0 0]  ProductsOfInertiaUnits=kg*m^2  GraphicType=FromGeometry  MarkerShape=Sphere  MarkerSize=10  GraphicVisPropType=SimpleVisualProperties  GraphicDiffuseColor=[0.6 0.0 0.0]  GraphicOpacity=1.0  GraphicSpecularColor=[0.5 0.5 0.5 1.0]  GraphicAmbientColor=[0.15 0.15 0.15 1.0]  GraphicEmissiveColor=[0.0 0.0 0.0 1.0]  GraphicShininess=75  DoExposeReferenceFrame=on  SerializedFrames=<Frames/>
  Ground : sm_lib/Body Elements/Brick Solid  BrickDimensions=[20 20 0.01]  BrickDimensionsUnits=m  ExportEntireGeometry=on  InertiaType=CalculateFromGeometry  BasedOnType=Density  Density=1000  DensityUnits=kg/m^3  Mass=1  MassUnits=kg  CenterOfMass=[0 0 0]  CenterOfMassUnits=m  MomentsOfInertia=[1 1 1]  MomentsOfInertiaUnits=kg*m^2  ProductsOfInertia=[0 0 0]  ProductsOfInertiaUnits=kg*m^2  GraphicType=FromGeometry  MarkerShape=Sphere  MarkerSize=10  GraphicVisPropType=SimpleVisualProperties  GraphicDiffuseColor=[1.0 1.0 1.0]  GraphicOpacity=1.0  GraphicSpecularColor=[0.5 0.5 0.5 1.0]  GraphicAmbientColor=[0.15 0.15 0.15 1.0]  GraphicEmissiveColor=[0.0 0.0 0.0 1.0]  GraphicShininess=75  DoExposeReferenceFrame=on  SerializedFrames=<Frames/>
  Ground frame : sm_lib/Frames and Transforms/World Frame
  Mechanism Configuration : sm_lib/Utilities/Mechanism Configuration  UniformGravity=Constant  GravityVector=[0 0 -9.80665]  GravityVectorUnits=m/s^2  LinearizationDelta=0.001  JointModeTransitionNonlinearIterations=2
  Rigid Transform1 : sm_lib/Frames and Transforms/Rigid Transform  RotationMethod=StandardAxis  FollAlignAxisA=+X  BaseAlignAxisA=+Y  FollAlignAxisB=+Y  BaseAlignAxisB=+Z  RotationStandardAxis=+X  RotationAngle=90  RotationAngleUnits=deg  RotationArbitraryAxis=[0 0 1]  RotationSequenceAxes=FollowerAxes  RotationSequence=XYX  RotationSequenceAngles=[0 0 0]  RotationSequenceAnglesUnits=deg  RotationMatrix=[1 0 0; 0 1 0; 0 0 1]  Quaternion=[1 0 0 0]  TranslationMethod=Cartesian  TranslationCartesianOffset=[0 0 -0.003]  TranslationCartesianOffsetUnits=m  TranslationStandardAxis=+Z  TranslationStandardOffset=0  TranslationStandardOffsetUnits=m  TranslationROffset=0  TranslationROffsetUnits=m  TranslationThetaOffset=0  TranslationThetaOffsetUnits=deg  TranslationZOffset=0  TranslationZOffsetUnits=m
  Rigid Transform2 : sm_lib/Frames and Transforms/Rigid Transform  RotationMethod=StandardAxis  FollAlignAxisA=+X  BaseAlignAxisA=+Y  FollAlignAxisB=+Y  BaseAlignAxisB=+Z  RotationStandardAxis=+Y  RotationAngle=90  RotationAngleUnits=deg  RotationArbitraryAxis=[0 0 1]  RotationSequenceAxes=FollowerAxes  RotationSequence=XYX  RotationSequenceAngles=[0 0 0]  RotationSequenceAnglesUnits=deg  RotationMatrix=[1 0 0; 0 1 0; 0 0 1]  Quaternion=[1 0 0 0]  TranslationMethod=Cartesian  TranslationCartesianOffset=[0.5 0 -0.003]  TranslationCartesianOffsetUnits=m  TranslationStandardAxis=+Z  TranslationStandardOffset=0  TranslationStandardOffsetUnits=m  TranslationROffset=0  TranslationROffsetUnits=m  TranslationThetaOffset=0  TranslationThetaOffsetUnits=deg  TranslationZOffset=0  TranslationZOffsetUnits=m
  Rigid Transform3 : sm_lib/Frames and Transforms/Rigid Transform  RotationMethod=None  FollAlignAxisA=+X  BaseAlignAxisA=+Y  FollAlignAxisB=+Y  BaseAlignAxisB=+Z  RotationStandardAxis=+Y  RotationAngle=90  RotationAngleUnits=deg  RotationArbitraryAxis=[0 0 1]  RotationSequenceAxes=FollowerAxes  RotationSequence=XYX  RotationSequenceAngles=[0 0 0]  RotationSequenceAnglesUnits=deg  RotationMatrix=[1 0 0; 0 1 0; 0 0 1]  Quaternion=[1 0 0 0]  TranslationMethod=Cartesian  TranslationCartesianOffset=[0 0 -0.003]  TranslationCartesianOffsetUnits=m  TranslationStandardAxis=+Z  TranslationStandardOffset=0  TranslationStandardOffsetUnits=m  TranslationROffset=0  TranslationROffsetUnits=m  TranslationThetaOffset=0  TranslationThetaOffsetUnits=deg  TranslationZOffset=0  TranslationZOffsetUnits=m
  Rigid Transform4 : sm_lib/Frames and Transforms/Rigid Transform  RotationMethod=StandardAxis  FollAlignAxisA=+X  BaseAlignAxisA=+Y  FollAlignAxisB=+Y  BaseAlignAxisB=+Z  RotationStandardAxis=+X  RotationAngle=90  RotationAngleUnits=deg  RotationArbitraryAxis=[0 0 1]  RotationSequenceAxes=FollowerAxes  RotationSequence=XYX  RotationSequenceAngles=[0 0 0]  RotationSequenceAnglesUnits=deg  RotationMatrix=[1 0 0; 0 1 0; 0 0 1]  Quaternion=[1 0 0 0]  TranslationMethod=Cartesian  TranslationCartesianOffset=[1 0 0.001]  TranslationCartesianOffsetUnits=m  TranslationStandardAxis=+Z  TranslationStandardOffset=0  TranslationStandardOffsetUnits=m  TranslationROffset=0  TranslationROffsetUnits=m  TranslationThetaOffset=0  TranslationThetaOffsetUnits=deg  TranslationZOffset=0  TranslationZOffsetUnits=m
  Rigid Transform5 : sm_lib/Frames and Transforms/Rigid Transform  RotationMethod=None  FollAlignAxisA=+X  BaseAlignAxisA=+Y  FollAlignAxisB=+Y  BaseAlignAxisB=+Z  RotationStandardAxis=+Z  RotationAngle=0.0  RotationAngleUnits=deg  RotationArbitraryAxis=[0 0 1]  RotationSequenceAxes=FollowerAxes  RotationSequence=XYX  RotationSequenceAngles=[0 0 0]  RotationSequenceAnglesUnits=deg  RotationMatrix=[1 0 0; 0 1 0; 0 0 1]  Quaternion=[1 0 0 0]  TranslationMethod=Cartesian  TranslationCartesianOffset=[0 0 -0.002]  TranslationCartesianOffsetUnits=m  TranslationStandardAxis=+Z  TranslationStandardOffset=0  TranslationStandardOffsetUnits=m  TranslationROffset=0  TranslationROffsetUnits=m  TranslationThetaOffset=0  TranslationThetaOffsetUnits=deg  TranslationZOffset=0  TranslationZOffsetUnits=m
  Rigid Transform6 : sm_lib/Frames and Transforms/Rigid Transform  RotationMethod=StandardAxis  FollAlignAxisA=+X  BaseAlignAxisA=+Y  FollAlignAxisB=+Y  BaseAlignAxisB=+Z  RotationStandardAxis=+X  RotationAngle=90  RotationAngleUnits=deg  RotationArbitraryAxis=[0 0 1]  RotationSequenceAxes=FollowerAxes  RotationSequence=XYX  RotationSequenceAngles=[0 0 0]  RotationSequenceAnglesUnits=deg  RotationMatrix=[1 0 0; 0 1 0; 0 0 1]  Quaternion=[1 0 0 0]  TranslationMethod=Cartesian  TranslationCartesianOffset=[2 0 0.001]  TranslationCartesianOffsetUnits=m  TranslationStandardAxis=+Z  TranslationStandardOffset=0  TranslationStandardOffsetUnits=m  TranslationROffset=0  TranslationROffsetUnits=m  TranslationThetaOffset=0  TranslationThetaOffsetUnits=deg  TranslationZOffset=0  TranslationZOffsetUnits=m
  Solver : nesl_utility/Solver Configuration  PhysicalDomain=network_engine_domain  SubClassName=solver  LeftPortType=input  RightPortType=generic  Tones=[]  Harmonics=[]  SimulateNoise=off  Profile=off  UseLocalSampling=off  EnableSwitchedLinearOptims=on  FrequencyDomain=off  UseCCode=off  RelTol=0.001  AbsTol=1e-06  MinStep=1e-09  ToWorkspace=off  RevertToSquareIcSolve=off  NumHomotopyIterations=100  PhasorMode=off  PhasorModeNumHarmonics=1  ConsistencySolver=NEWTON_XTOL_AFTER_FTOL  CanonicalOrdering=UNORDERED  OptimizeIntermediates=UNOPTIMIZED  IndexReductionMethod=DerivativeReplacement  DoDC=off  ResidualTolerance=1e-09  ConsistencyTolSource=GLOBAL  ConsistencyAbsTol=0.001  ConsistencyRelTol=0.001  ConsistencyTolFactor=0.001  UseLocalSolver=off  LocalSolverChoice=NE_BACKWARD_EULER_ADVANCER  ResolveIndetEquations=on  FunctionEvalNumThread=1  LocalSolverSampleTime=0.001  DoFixedCost=off  MaxNonlinIter=3  MaxModeIter=2  ComputeImpulses=off  ImpulseIterations=2  LinearAlgebra=Sparse  LinearAlgebraNumThread=0  EquationFormulation=NE_TIME_EF  DelaysMemoryBudget=1024  AutomaticFiltering=on  FilteringTimeConstant=0.001  PartitionStorageMethod=AS_NEEDED  PartitionMemoryBudget=1024  PartitionMethod=FAST  MultibodyUseLocalSolver=off  MultibodyLocalSolverChoice=ODE1  MultibodyLocalSolverSampleTime=0.001
  surface : PMIOPort  Side=Left
  Origo : PMIOPort  Port=2  Side=Left
  connections:
  Ground frame/RConn1 -- Origo/RConn1 -- Rigid Transform5/LConn1 -- Solver/RConn1 -- Mechanism Configuration/RConn1
  Cylindrical Solid1/RConn1 -- Rigid Transform2/RConn1
  surface/RConn1 -- Ground/LConn1
  Cylindrical Solid/RConn1 -- Rigid Transform1/RConn1
  Rigid Transform5/RConn1 -- Rigid Transform3/LConn1 -- Rigid Transform6/LConn1 -- Rigid Transform4/LConn1 -- Rigid Transform1/LConn1 -- Rigid Transform2/LConn1
  Rigid Transform3/RConn1 -- Ground/RConn1
  Cylindrical Solid2/RConn1 -- Rigid Transform4/RConn1
  Cylindrical Solid3/RConn1 -- Rigid Transform6/RConn1
